simulink model "gas_mnist_base"  (R2017a)
settings: Solver=VariableStepAuto  StartTime=0.0  StopTime=10.0  RelTol=1e-3
libraries: ad_blocks x8
settings Model: Creator=percro2  LastModifiedBy=percro2

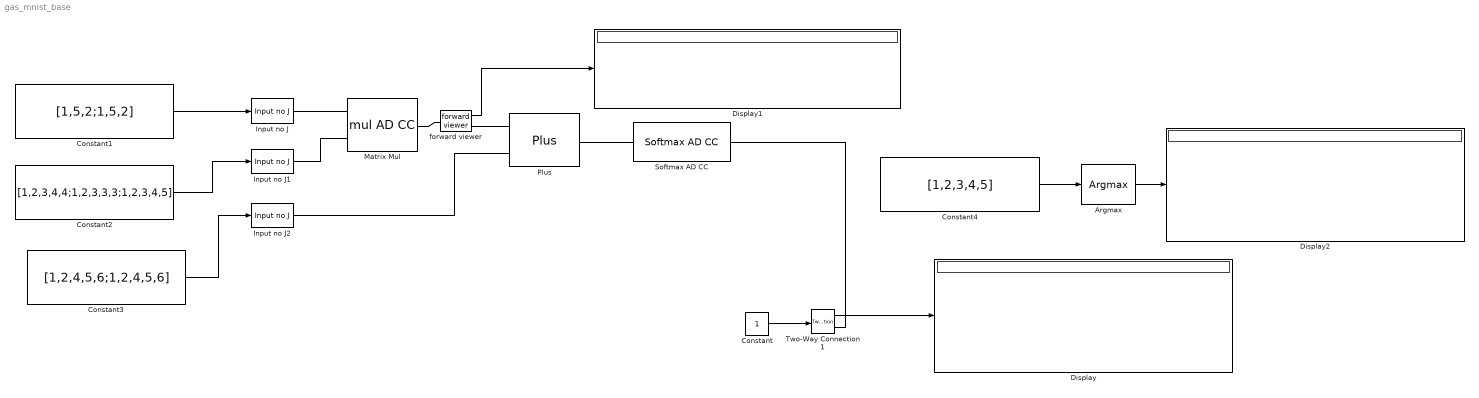
== system gas_mnist_base ==
  "Argmax " : ad_blocks/Argmax   dim=1
  Constant : Constant
  Constant1 : Constant  Value=[1,5,2;1,5,2]  VectorParams1D=off
  Constant2 : Constant  Value=[1,2,3,4,4;1,2,3,3,3;1,2,3,4,5]  VectorParams1D=off
  Constant3 : Constant  Value=[1,2,4,5,6;1,2,4,5,6]  VectorParams1D=off
  Constant4 : Constant  Value=[1,2,3,4,5]  VectorParams1D=off
  Display : Display
  Display1 : Display
  Display2 : Display
  Input no J : ad_blocks/Input no J  SystemSampleTime=-1
  Input no J1 : ad_blocks/Input no J  SystemSampleTime=-1
  Input no J2 : ad_blocks/Input no J  SystemSampleTime=-1
  Matrix Mul : ad_blocks/mul AD CC
  Plus : ad_blocks/Plus
  Softmax AD CC : ad_blocks/Softmax AD CC  SystemSampleTime=-1
  Two-Way Connection1 : TwoWayConnection
  forward viewer : ad_blocks/forward viewer  SystemSampleTime=-1
  wires:
  Constant1/1 -> Input no J/1
  Constant/1 -> Two-Way Connection1/1
  Two-Way Connection1/1 -> Display/1
  Constant2/1 -> Input no J1/1
  Constant3/1 -> Input no J2/1
  forward viewer/1 -> Display1/1
  Constant4/1 -> "Argmax "/1
  "Argmax "/1 -> Display2/1
  connections:
  Softmax AD CC/LConn1 -- Plus/RConn1
  Input no J2/RConn1 -- Plus/LConn2
  Input no J1/RConn1 -- Matrix Mul/LConn2
  Input no J/RConn1 -- Matrix Mul/LConn1
  Matrix Mul/RConn1 -- forward viewer/LConn1
  forward viewer/RConn1 -- Plus/LConn1
  Two-Way Connection1/RConn1 -- Softmax AD CC/RConn1
